simulink model "buck_05_2018_b"  (Simulink 9.2)
settings: Solver=ode45  StartTime=0.0  StopTime=2000/F  MaxStep=1/(10*F)  RelTol=1e-3  EnableMultiTasking=on
values from neighbouring files (symbols this model uses):
  C = 9.3e-6    (= 9.3e-06)    [buck_01_script.m]    (also in buck_02_script.m; buck_04_script.m)
  C1 = 5.5e-6    (= 5.5e-06)    [buck_01_script.m]    (also in buck_02_script.m; buck_04_script.m)
  Kp = 10^(-50/20)    (= 0.00316227766017)    [buck_04_script.m]
  L = 1.9e-6    (= 1.9e-06)    [buck_01_script.m]    (also in buck_02_script.m; buck_04_script.m)
  L1 = 5e-6    (= 5e-06)    [buck_01_script.m]    (also in buck_02_script.m; buck_04_script.m)
  R = Vs^2 / Ps    (= 5.445)    [buck_01_script.m]    (also in buck_02_script.m = 0.5445; buck_04_script.m)
  Ti = 1e-6    (= 1e-06)    [buck_04_script.m]
  Ve = 5    [buck_01_script.m]    (also in buck_02_script.m; buck_04_script.m)
  Vs = 3.3    [buck_01_script.m]    (also in buck_02_script.m; buck_04_script.m)
undefined symbols (not defined in the file or in its folder): powergui
libraries: powerlib x15, simulink x1
settings Model: Creator=lefrancp  LastModifiedBy=lefrancp
settings DataIOCC: SaveFinalState=on  SignalLoggingSaveFormat=Dataset  SaveOutput=off
settings DebuggingCC: UnderspecifiedInitializationDetection=Simplified  MergeDetectMultiDrivingBlocksExec=error  SolverPrmCheckMsg=warning  FcnCallInpInsideContextMsg=error  StateNameClashWarn=none
settings GRTTargetCC: CombineOutputUpdateFcns=on  GRTInterface=off
settings ConfigComp: CovSFcnEnable=off
settings SimscapeCC: SimscapeNormalizeSystem=off

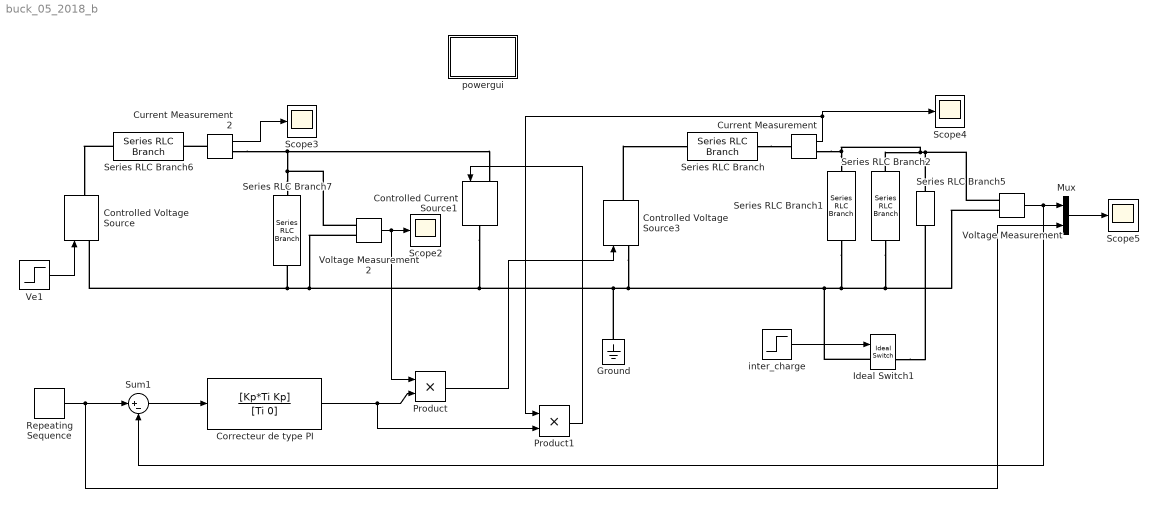
== system buck_05_2018_b ==
  Controlled Current Source1 : powerlib/Electrical Sources/Controlled Current Source  Initialize=on  Source_Type=AC  Amplitude=0  Phase=0  Frequency=0  Measurements=None
  Controlled Voltage Source : powerlib/Electrical Sources/Controlled Voltage Source  Initialize=on  Source_Type=AC  Amplitude=0  Phase=0  Frequency=0  Measurements=None
  Controlled Voltage Source3 : powerlib/Electrical Sources/Controlled Voltage Source  Initialize=on  Source_Type=AC  Amplitude=0  Phase=0  Frequency=0  Measurements=None
  Correcteur de type PI : TransferFcn  Numerator=[Kp*Ti Kp]  Denominator=[Ti 0]
  Current Measurement : powerlib/Measurements/Current Measurement  PhasorSimulation=off  OutputType=Complex  PSBequivalent=0
  Current Measurement2 : powerlib/Measurements/Current Measurement  PhasorSimulation=off  OutputType=Complex  PSBequivalent=0
  Ground : powerlib/Elements/Ground  LConnTagsString=a
  Ideal Switch1 : powerlib/Power Electronics/Ideal Switch  Ron=0.001  Lon=0  IC=0  Rs=1e5  Cs=inf  Measurements=on
  Mux : Mux  Inputs=2
  Product : Product
  Product1 : Product
  Repeating Sequence : simulink/Sources/Repeating Sequence  rep_seq_t=[0 1e-3 10e-3]  rep_seq_y=[0 Vs Vs]
  Scope{2..5} (4 alike) : Scope
  Series RLC Branch : powerlib/Elements/Series RLC Branch  LConnTagsString=__new0  RConnTagsString=__new0  BranchType=L  Resistance=1  Inductance=L  SetiL0=off  InitialCurrent=0  Capacitance=1e-6  Setx0=off  InitialVoltage=0  Measurements=None
  Series RLC Branch1 : powerlib/Elements/Series RLC Branch  LConnTagsString=__new0  RConnTagsString=__new0  BranchType=C  Resistance=1  Inductance=L  SetiL0=off  InitialCurrent=0  Capacitance=C  Setx0=off  InitialVoltage=0  Measurements=None
  Series RLC Branch2 : powerlib/Elements/Series RLC Branch  LConnTagsString=__new0  RConnTagsString=__new0  BranchType=R  Resistance=R  Inductance=L  SetiL0=off  InitialCurrent=0  Capacitance=C  Setx0=off  InitialVoltage=0  Measurements=None
  Series RLC Branch5 : powerlib/Elements/Series RLC Branch  LConnTagsString=__new0  RConnTagsString=__new0  BranchType=R  Resistance=R*10  Inductance=L  SetiL0=off  InitialCurrent=0  Capacitance=C  Setx0=off  InitialVoltage=0  Measurements=None
  Series RLC Branch6 : powerlib/Elements/Series RLC Branch  LConnTagsString=__new0  RConnTagsString=__new0  BranchType=L  Resistance=1  Inductance=L1  SetiL0=off  InitialCurrent=0  Capacitance=1e-6  Setx0=off  InitialVoltage=0  Measurements=None
  Series RLC Branch7 : powerlib/Elements/Series RLC Branch  LConnTagsString=__new0  RConnTagsString=__new0  BranchType=C  Resistance=1  Inductance=L  SetiL0=off  InitialCurrent=0  Capacitance=C1  Setx0=off  InitialVoltage=0  Measurements=None
  Sum1 : Sum  Inputs=|+-
  Ve1 : Step  Time=2e-3  Before=Ve  After=Ve+0.1  SampleTime=0
  Voltage Measurement : powerlib/Measurements/Voltage Measurement  PhasorSimulation=off  OutputType=Complex  PSBequivalent=0
  Voltage Measurement2 : powerlib/Measurements/Voltage Measurement  PhasorSimulation=off  OutputType=Complex  PSBequivalent=0
  inter_charge : Step  Time=3e-3  SampleTime=0
  powergui : Subsystem  Priority=1  AncestorBlock=powerlib/powergui  DialogController=POWERSYS.PowerSysDialog  InitFcn=powergui( 'InitFcn_Callback' , gcb , 0 , [ ] );  mask(PSB option menu block){SimulationMode=Continuous, SampleTime=50e-6, frequency=60, Iterations=50, frequencyindice=0, Pbase=100e6, ErrMax=1e-4, UnitsV=kV, UnitsW=MW, buscounter=0, FunctionMessages=off, echomessages=off, EnableUseOfTLC=off, CurrentSourceSwitches=on, DisableSnubberDevices=off, DisableRonSwitches=off, DisableVfSwitches=off, DisplayEquations=off, AutomaticDiscreteSolvers=off, SolverType=Tustin, Interpol=off, ExternalGateDelay=off, methode=off, Ts=0, x0status=blocks, SPID=off, SwTol=0, HookPort=off, NonlinearTolerance=0, nMaxIteration=15, ContinueOnMaxIteration=off, RestoreLinks=warning, ResistiveCurrentMeasurement=off, Frange=[0:2:500], Ylog=off, Xlog=on, ShowGrid=off, save=off, variable=ZData, structure=0, ZoomFFT=off, StartTime=0.0, cycles=1, DisplayStyle=1, fundamental=60, FreqAxis=off, MaxFrequency=1000, frequencyindicesteady=1, RmsSteady=1, display=off}
      mask prompts: SimulationMode "Simulation type:"; SampleTime "Sample time (s):"; frequency "Frequency (Hz):"; Iterations "Max iterations"; frequencyindice "Frequency (Hz)"; Pbase "Base power (VA)"; ErrMax "PQ tolerance (pu)"; UnitsV "Voltage units"; UnitsW "Power units"; buscounter "Load flow bus counter"; FunctionMessages "Disable Specialized Power Systems warnings"; echomessages "Display Specialized Power Systems compilation messages"; EnableUseOfTLC "Use TLC file when in Accelerator Simulation Mode and for code generation"; CurrentSourceSwitches "Disable ideal switching"; DisableSnubberDevices "Disable snubbers in switching devices"; DisableRonSwitches "Disable Ron resistances in switching devices"; DisableVfSwitches "Disable forward voltages in switching devices"; DisplayEquations "Display circuit differential equations"; AutomaticDiscreteSolvers "Automatically handle Discrete solver and Advanced tab solver settings of blocks"; SolverType "Discrete solver"; Interpol "Interpolate switching events"; ExternalGateDelay "Use time-stamped gate signals"; methode "Store switching topologies"; Ts "Buffer size (MBytes):"; x0status "Start simulation with initial electrical states from:"; SPID "Use ideal switching devices"; SwTol "Switch tolerance"; HookPort "Allow multiple powergui blocks"; NonlinearTolerance "Solver tolerance"; nMaxIteration "Maximum number of iterations"; ContinueOnMaxIteration "Continue Simulation if maximum number of iterations is reached"; RestoreLinks "Restore disabled links of Simscape Power Systems ST blocks:"; ResistiveCurrentMeasurement "Use non ideal current measurement blocks (1e-4Ohm internal resistance)"; Frange "Frequency Range"; Ylog "Log impedance"; Xlog "log Frequency"; ShowGrid "grid"; save "Save Data To Workspace"; variable "Variable Name"; structure "Structure Name (PSBFFTSCOPE)"; ZoomFFT "ZoomFFT (PSBFFTSCOPE)"; StartTime "Start Time (PSBFFTSCOPE)"; cycles "Cycles (PSBFFTSCOPE)"; DisplayStyle "Display style (PSBFFTSCOPE)"; fundamental "Fundamental (PSBFFTSCOPE)"; FreqAxis "Frequency Axis (PSBFFTSCOPE)"; MaxFrequency "Max Frequency (PSBFFTSCOPE)"; frequencyindicesteady "Frequency indice (STEADYSTATE)"; RmsSteady "RMS display (STEADYSTATE)"; display "Display Results"
      mask help: Set simulation type, simulation parameters, and preferences.
      mask init:
      | dispMessage = powergui('MaskInitialization',gcb,SimulationMode,SampleTime);
      settings: PreSaveFcn=powergui( 'PreSaveFcn_Callback' , gcb , [ ] , [ ] );  OpenFcn=sps_rtmsupport('OpenFcn',gcbh)
      mask Help: helpview(psbhelp)
      mask TypeOptions SimulationMode: Continuous | Discrete | Phasor | Discrete phasor
      mask Callback SimulationMode: powergui('SimulationType',[],[],gcb);
      mask TypeOptions UnitsV: V | kV
      mask TypeOptions UnitsW: W | kW | MW
      mask Callback CurrentSourceSwitches: powergui('SimulationType',[],[],gcb);
      mask Callback AutomaticDiscreteSolvers: powergui('SimulationType',[],[],gcb);
      mask TypeOptions SolverType: Tustin/Backward Euler (TBE) | Tustin | Backward Euler
      mask Callback SolverType: powergui('SimulationType',[],[],gcb);
      mask Callback Interpol: powergui('SimulationType',[],[],gcb);
      mask Callback ExternalGateDelay: powergui('SimulationType',[],[],gcb);
      mask Callback methode: powergui('SimulationType',[],[],gcb);
      mask TypeOptions x0status: blocks | steady | zero
      mask TypeOptions RestoreLinks: yes | warning | no
      mask Callback display: sps_rtmsupport('parametereditingmodes',gcbh) % Will be executed last in parameter callbacks to ensure mask enable consistency
      mask Callback RLCLineParameters:
      | close_system(gcb)
      | powerLineParameters
      mask Callback DecouplingLines:
      | close_system(gcb);
      | DecouplingLineReplace(gcs)
      mask DialogControl AutoSolverNote Prompt: The Simulation type parameter is governed by Simulink. To access the Powergui solver settings, unselect auto (Automatic solver selection) solver in the Simulink solver options.
      mask DialogControl SteadyState Prompt: Steady-State
      mask DialogControl SteadyState Callback:
      | close_system(gcb)
      | power_steadystate(bdroot(gcb),gcb);
      mask DialogControl InitialState Prompt: Initial State
      mask DialogControl InitialState Callback:
      | close_system(gcb)
      | power_initstates(bdroot(gcb),gcb)
      mask DialogControl MachineInitialization Prompt: Machine Initialization
      mask DialogControl MachineInitialization Callback:
      | close_system(gcb)
      | power_loadflow(bdroot(gcb),gcb)
      mask DialogControl ImpedanceMeasurement Prompt: Impedance Measurement
      mask DialogControl ImpedanceMeasurement Callback:
      | close_system(gcb)
      | power_zmeter(bdroot(gcb),gcb)
      mask DialogControl RLCLineParametersButton Prompt: RLC Line Parameters *
      mask DialogControl RLCLineParametersButton Tooltip: * The power_lineparam function is now accessible only from the command line.
      mask DialogControl Control16 Prompt: * The power_lineparam function is now accessible only from the command line. The Compute Line Parameters App can be used. See the power_lineparam documentation for more informations
      mask DialogControl FFTAnalysis Prompt: FFT Analysis
      mask DialogControl FFTAnalysis Callback:
      | close_system(gcb)
      | power_fftscope(bdroot(gcb),gcb)
      mask DialogControl LinearSystemAnalyzer Prompt: Use Linear System Analyzer
      mask DialogControl LinearSystemAnalyzer Callback:
      | close_system(gcb)
      | power_ltiview(bdroot(gcb),gcb)
      mask DialogControl HysteresisDesign Prompt: Hysteresis Design
      mask DialogControl HysteresisDesign Callback:
      | close_system(gcb)
      | power_hysteresis(bdroot(gcb),gcb)
      mask DialogControl GenerateReprot Prompt: Generate Report
      mask DialogControl GenerateReprot Callback:
      | close_system(gcb)
      | power_report(bdroot(gcb),gcb)
      mask DialogControl Control14 Prompt: Customize SPS blocks
      mask DialogControl Control14 Callback:
      | close_system(gcb);
      | power_customize;
      mask DialogControl LoadFlow Prompt: Load Flow
      mask DialogControl LoadFlow Callback:
      | close_system(gcb)
      | power_loadflow('-v2',bdroot(gcb))
      mask DialogControl Container14 Prompt: Load flow settings
      mask DialogControl Solver Prompt: Solver
      mask DialogControl SolverDetails Prompt: Solver details for nonlinear elements
      mask Display: color('blue'),disp(dispMessage)
  wires:
  Voltage Measurement/1 -> Sum1/2, Mux/1
  Current Measurement/1 -> Product1/1, Scope4/1
  Ve1/1 -> Controlled Voltage Source/1
  Voltage Measurement2/1 -> Product/1, Scope2/1
  Current Measurement2/1 -> Scope3/1
  Correcteur de type PI/1 -> Product1/2, Product/2
  Product/1 -> Controlled Voltage Source3/1
  Product1/1 -> Controlled Current Source1/1
  Repeating Sequence/1 -> Mux/2, Sum1/1
  Sum1/1 -> Correcteur de type PI/1
  inter_charge/1 -> Ideal Switch1/1
  Mux/1 -> Scope5/1
  connections:
  Ground/LConn1 -- Ideal Switch1/LConn1 -- Series RLC Branch1/RConn1 -- Voltage Measurement/LConn2 -- Series RLC Branch2/RConn1 -- Controlled Voltage Source3/LConn1 -- Controlled Current Source1/RConn1 -- Voltage Measurement2/LConn2 -- Series RLC Branch7/RConn1 -- Controlled Voltage Source/LConn1
  Controlled Voltage Source3/RConn1 -- Series RLC Branch/LConn1
  Series RLC Branch1/LConn1 -- Current Measurement/RConn1 -- Series RLC Branch5/LConn1 -- Voltage Measurement/LConn1 -- Series RLC Branch2/LConn1
  Series RLC Branch7/LConn1 -- Voltage Measurement2/LConn1 -- Controlled Current Source1/LConn1 -- Current Measurement2/RConn1
  Series RLC Branch/RConn1 -- Current Measurement/LConn1
  Series RLC Branch6/LConn1 -- Controlled Voltage Source/RConn1
  Current Measurement2/LConn1 -- Series RLC Branch6/RConn1
  Ideal Switch1/RConn1 -- Series RLC Branch5/RConn1

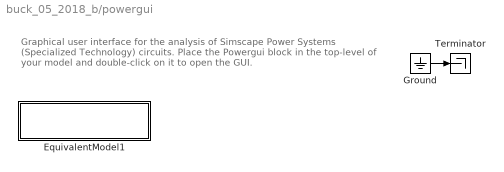
== system buck_05_2018_b/powergui ==
  note: Graphical user interface for the analysis of
      | Simscape Power Systems (Specialized Technology) circuits.
      | Place the Powergui block in the top-level of your model and double-click
      | on it to open the GUI.
  EquivalentModel1 : Subsystem
      mask init:
      | S  = GetDataForEquivalentModel('Continuous',gcbh);
      mask Display:
      | color('blue')
      | disp('EQUIVALENT CIRCUIT\nContinuous')
      | disp('')
  Ground : Ground
  Terminator : Terminator
  wires:
  Ground/1 -> Terminator/1

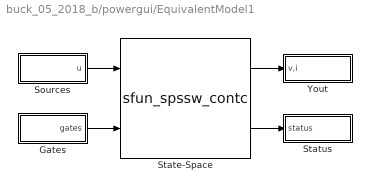
== system buck_05_2018_b/powergui/EquivalentModel1 ==
  Gates : Subsystem
  Sources : Subsystem
  State-Space : S-Function  FunctionName=sfun_spssw_contc  Parameters=S.A, S.B, S.C, S.D, S.x0, S.EnableUseOfTLC,S.SwitchResistance ,S.SwitchType, S.SwitchGateInitialValue, S.OutputsToResetToZero,S.SaveMatrices,S.BufferSize  SFunctionDeploymentMode=off  EnableBusSupport=off
  Status : Subsystem
  Yout : Subsystem
  wires:
  Gates/1(gates) -> State-Space/2
  Sources/1(u) -> State-Space/1
  State-Space/2 -> Status/1(status)
  State-Space/1 -> Yout/1(v,i)

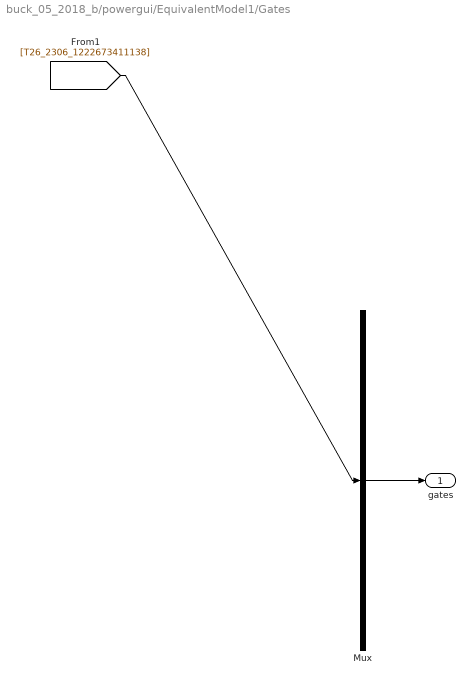
== system buck_05_2018_b/powergui/EquivalentModel1/Gates ==
  Mux : Mux  Inputs=1
  gates : Outport  VectorParamsAs1DForOutWhenUnconnected=off
  wires:
  Mux/1 -> gates/1
  [T26_2306_1222673411138] -> Mux/1

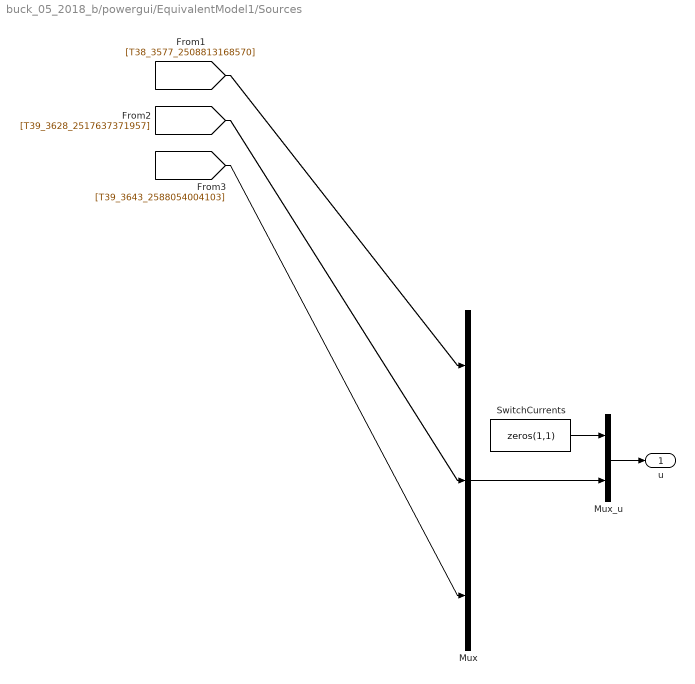
== system buck_05_2018_b/powergui/EquivalentModel1/Sources ==
  Mux : Mux  Inputs=[1 1 1]
  Mux_u : Mux  Inputs=[1 3]
  SwitchCurrents : Constant  Value=zeros(1,1)
  u : Outport  VectorParamsAs1DForOutWhenUnconnected=off
  wires:
  Mux/1 -> Mux_u/2
  SwitchCurrents/1 -> Mux_u/1
  Mux_u/1 -> u/1
  [T38_3577_2508813168570] -> Mux/1
  [T39_3628_2517637371957] -> Mux/2
  [T39_3643_2588054004103] -> Mux/3

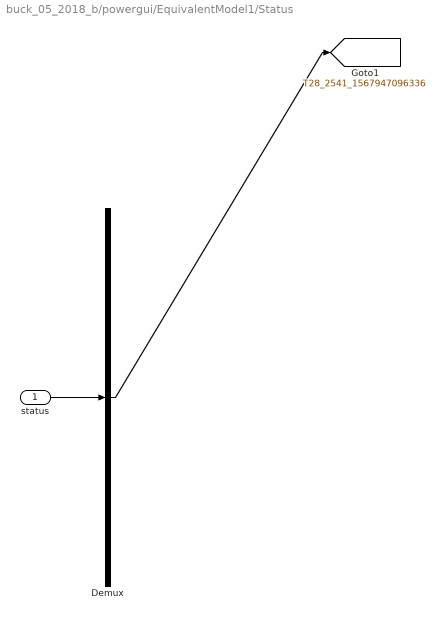
== system buck_05_2018_b/powergui/EquivalentModel1/Status ==
  status : Inport
  Demux : Demux  Outputs=1
  tag scope: T28_2541_1567947096336=global
  wires:
  status/1 -> Demux/1
  Demux/1 -> [T28_2541_1567947096336]

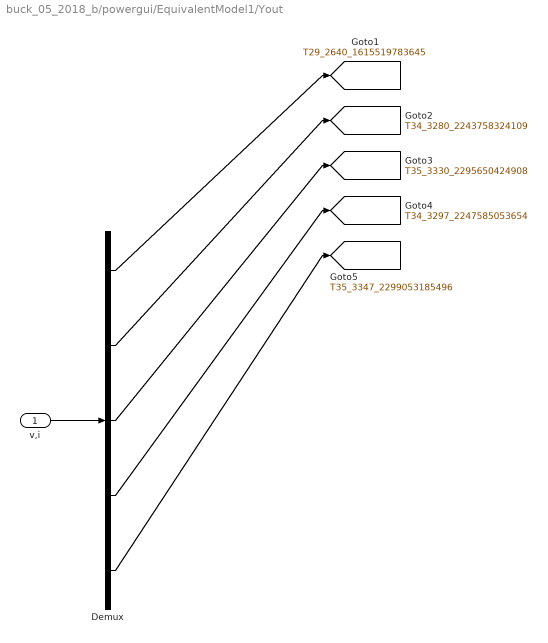
== system buck_05_2018_b/powergui/EquivalentModel1/Yout ==
  v,i : Inport
  Demux : Demux  Outputs=[1 1 1 1 1]
  tag scope: T29_2640_1615519783645=global, T34_3280_2243758324109=global, T34_3297_2247585053654=global, T35_3330_2295650424908=global, T35_3347_2299053185496=global
  wires:
  v,i/1 -> Demux/1
  Demux/1 -> [T29_2640_1615519783645]
  Demux/2 -> [T34_3280_2243758324109]
  Demux/3 -> [T35_3330_2295650424908]
  Demux/4 -> [T34_3297_2247585053654]
  Demux/5 -> [T35_3347_2299053185496]
